simulink model "ls_legolabs"  (R2024b)
settings: Solver=FixedStepAuto  StartTime=0.0  StopTime=10.0  RelTol=1e-3  EnableMultiTasking=on
libraries: legoev3lib x14, simulink x1
settings Model: ExtModeTrigDuration=2  Creator=eline.schjerven  LastModifiedBy=seyon
settings SolverCC: PositivePriorityOrder=on
settings OptimizationCC: EnhancedBackFolding=on  PassReuseOutputArgsThreshold=0  MaxStackSize=64  OptimizeBlockOrder=speed  DifferentSizesBufferReuse=on  OptimizationCustomize=off
settings DebuggingCC: ParameterTunabilityLossMsg=error
settings HardwareCC: ProdBitPerPointer=32  ProdBitPerSizeT=32  ProdBitPerPtrDiffT=32  ProdLargestAtomicInteger=Long  ProdWordSize=32  ProdHWDeviceType=ARM Compatible->ARM 9  UseEmbeddedCoderFeatures=off  UseSimulinkCoderFeatures=off
settings SFSimCC: MATLABDynamicMemAlloc=off
settings RTWCC: Description=Embedded Coder  SystemTargetFile=ert.tlc  HardwareBoard=LEGO MINDSTORMS EV3  TLCOptions="-aInlineSetEventsForThisBaseRateFcn=TLC_FALSE -aSuppressMultiTaskScheduler=TLC_FALSE  -aRateBasedStepFcn=0"  TemplateMakefile=ert_default_tmf  Toolchain=Sourcery G++ Lite v2009q3
settings CodeAppCC: ForceParamTrailComments=on  OperatorAnnotations=on
settings ERTTargetCC: ERTCustomFileBanners=off  SupportContinuousTime=on  SupportNonInlinedSFcns=on  RemoveResetFunc=off  SupportVariableSizeSignals=on  ModelStepFunctionPrototypeControlCompliant=off  ExtModeTransport=2  ExtModeStaticAlloc=on  ExtModeMexFile=ext_xcp  ExtModeIntrfLevel=Level2 - Open  InlinedParameterPlacement=Hierarchical  DynamicArrayContainerType=coder::array

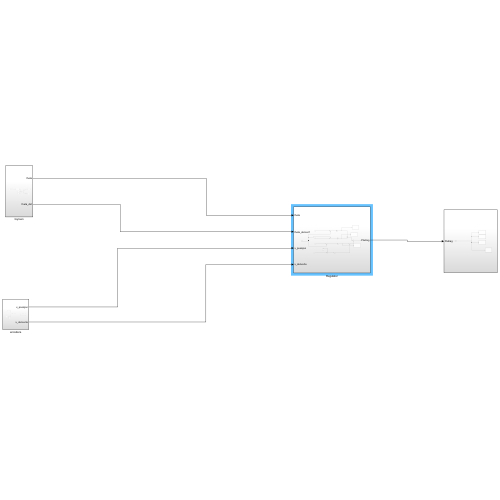
[thumbnail: Simulink's stored preview of the top-level diagram]
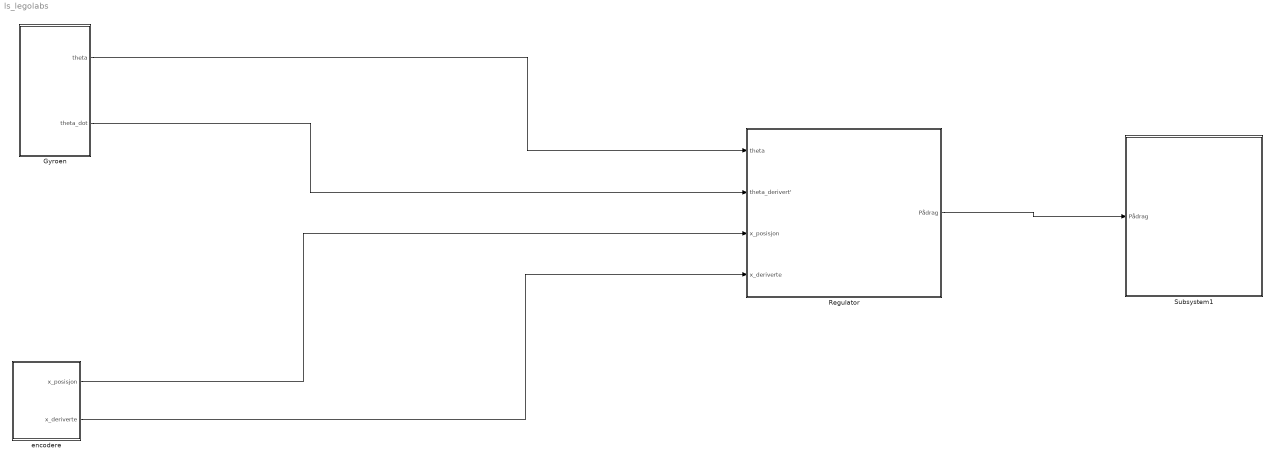
== system ls_legolabs ==
  Gyroen : Subsystem
  Regulator : Subsystem
  Subsystem1 : Subsystem
  encodere : Subsystem
  wires:
  Gyroen/2(theta_dot) -> Regulator/2(theta_derivert')
  encodere/1(x_posisjon) -> Regulator/3(x_posisjon)
  Gyroen/1(theta) -> Regulator/1(theta)
  encodere/2(x_deriverte) -> Regulator/4(x_deriverte)
  Regulator/1(Pådrag) -> Subsystem1/1(Pådrag)

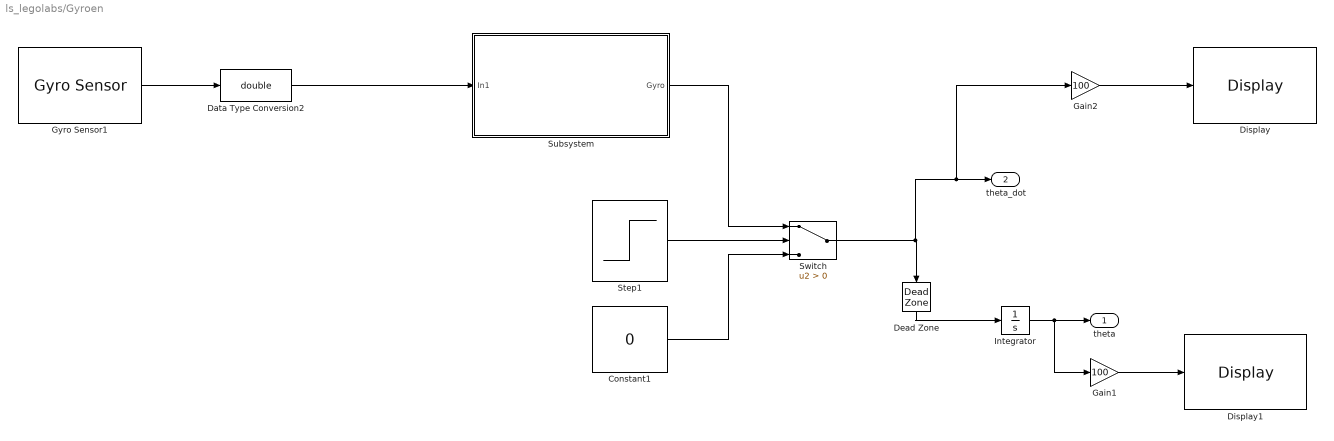
== system ls_legolabs/Gyroen ==
  Constant1 : Constant  Value=0
  Data Type Conversion2 : DataTypeConversion  OutDataTypeStr=double  SaturateOnIntegerOverflow=off  RndMeth=Floor
  Dead Zone : DeadZone  LowerValue=-1  UpperValue=1
  Display : legoev3lib/Display  slcdStr=tet_dev  slcdLine=1  slcdFormat=Decimal
  Display1 : legoev3lib/Display  slcdStr=tet  slcdLine=2  slcdFormat=Decimal
  Gain1 : Gain  Gain=100
  Gain2 : Gain  Gain=100
  Gyro Sensor1 : legoev3lib/Gyro Sensor  portNumber=2  sampleTime=0.01
  Integrator : Integrator
  Step1 : Step  Time=5  SampleTime=0
  Subsystem : Subsystem
  Switch : Switch  Criteria=u2 > Threshold  SaturateOnIntegerOverflow=off  InputSameDT=off
  theta : Outport
  theta_dot : Outport  Port=2
  wires:
  Integrator/1 -> Gain1/1, theta/1
  Gyro Sensor1/1 -> Data Type Conversion2/1
  Data Type Conversion2/1 -> Subsystem/1(In1)
  Step1/1 -> Switch/2
  Subsystem/1(Gyro) -> Switch/1
  Constant1/1 -> Switch/3
  Switch/1 -> Dead Zone/1, Gain2/1, theta_dot/1
  Gain1/1 -> Display1/1
  Gain2/1 -> Display/1
  Dead Zone/1 -> Integrator/1

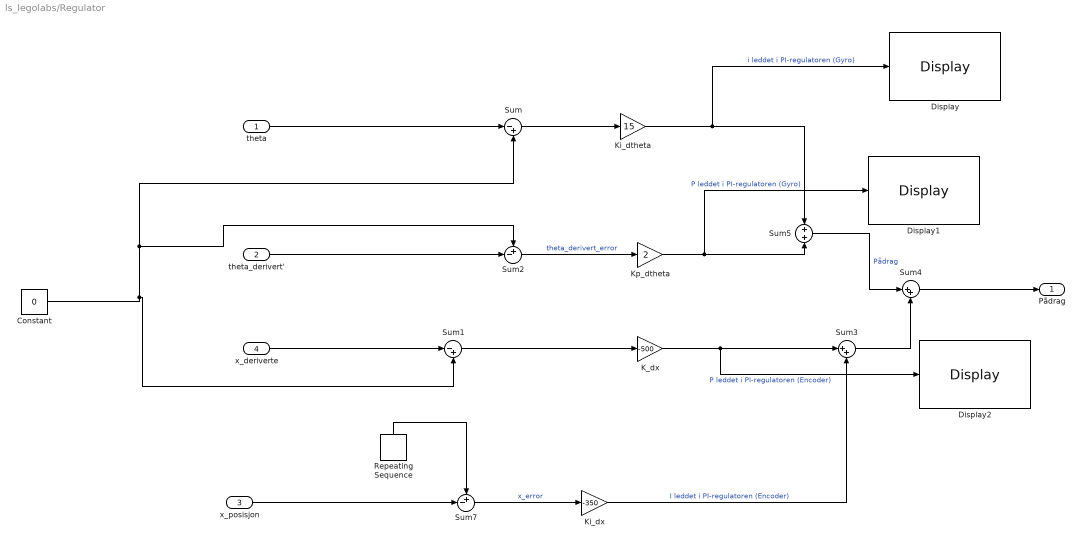
== system ls_legolabs/Regulator ==
  theta : Inport
  theta_derivert' : Inport  Port=2
  x_posisjon : Inport  Port=3
  x_deriverte : Inport  Port=4
  Constant : Constant  Value=0
  Display : legoev3lib/Display  slcdStr=Ti_I  slcdLine=9  slcdFormat=Decimal
  Display1 : legoev3lib/Display  slcdStr=Tp_dt  slcdLine=10  slcdFormat=Decimal
  Display2 : legoev3lib/Display  slcdStr=Kp_dx  slcdLine=8  slcdFormat=Decimal
  K_dx : Gain  Gain=-500
  Ki_dtheta : Gain  Gain=15
  Ki_dx : Gain  Gain=-350
  Kp_dtheta : Gain  Gain=2
  Repeating Sequence : simulink/Sources/Repeating Sequence  rep_seq_t=[0 5 7 10 12 14 16 1000]  rep_seq_y=[0 0 0.25 0.4 0.8 1.0 1.2 1.2]
  Sum : Sum  Inputs=|-+
  Sum1 : Sum  Inputs=|-+
  Sum2 : Sum  Inputs=+-|
  Sum3 : Sum  Inputs=|++
  Sum4 : Sum  Inputs=|++
  Sum5 : Sum
  Sum7 : Sum  Inputs=+-|
  Pådrag : Outport
  wires:
  Kp_dtheta/1 -> Sum5/2, Display1/1  "P leddet i PI-regulatoren (Gyro)"
  K_dx/1 -> Display2/1, Sum3/1  "P leddet i PI-regulatoren (Encoder)"
  Ki_dtheta/1 -> Display/1, Sum5/1  "i leddet i PI-regulatoren (Gyro)"
  theta_derivert'/1 -> Sum2/2
  x_posisjon/1 -> Sum7/2
  Ki_dx/1 -> Sum3/2  "I leddet i PI-regulatoren (Encoder)"
  Sum7/1 -> Ki_dx/1  "x_error"
  Sum2/1 -> Kp_dtheta/1  "theta_derivert_error"
  Sum/1 -> Ki_dtheta/1
  theta/1 -> Sum/1
  Constant/1 -> Sum1/2, Sum2/1, Sum/2
  x_deriverte/1 -> Sum1/1
  Sum1/1 -> K_dx/1
  Sum3/1 -> Sum4/2
  Sum5/1 -> Sum4/1  "Pådrag"
  Sum4/1 -> Pådrag/1
  Repeating Sequence/1 -> Sum7/1

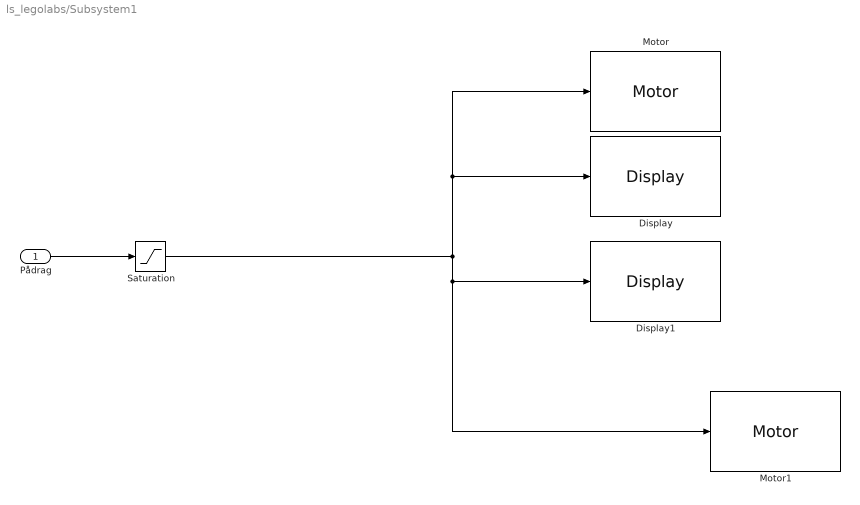
== system ls_legolabs/Subsystem1 ==
  Pådrag : Inport
  Display : legoev3lib/Display  slcdStr=Motor B  slcdLine=3  slcdFormat=Decimal
  Display1 : legoev3lib/Display  slcdStr=Motor C  slcdLine=4  slcdFormat=Decimal
  Motor : legoev3lib/Motor  sportNumber=C  sstopAction=Brake
  Motor1 : legoev3lib/Motor  sportNumber=B  sstopAction=Brake
  Saturation : Saturate  UpperLimit=100  LowerLimit=-100
  wires:
  Pådrag/1 -> Saturation/1
  Saturation/1 -> Motor1/1, Display1/1, Display/1, Motor/1

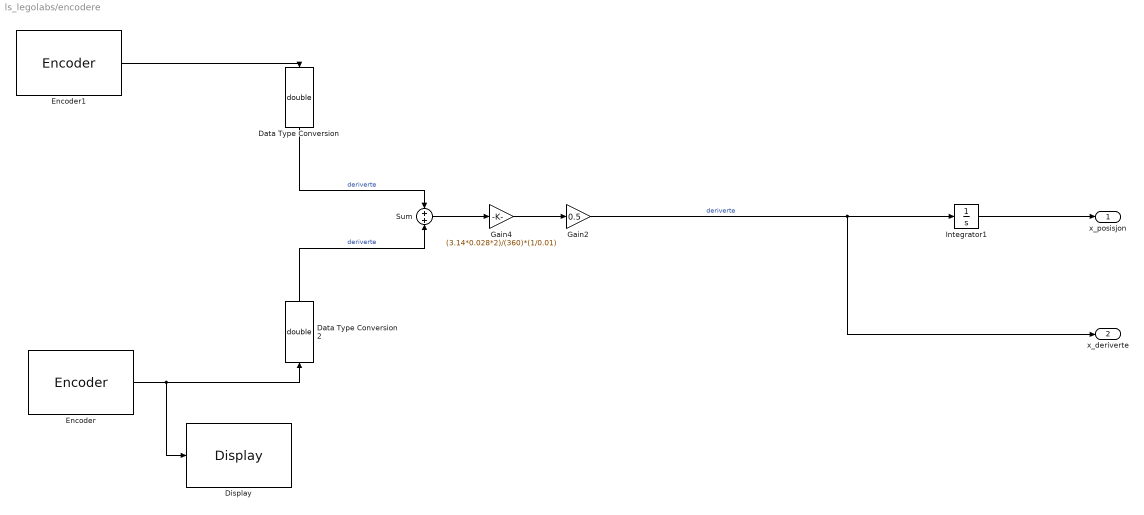
== system ls_legolabs/encodere ==
  Data Type Conversion : DataTypeConversion  OutDataTypeStr=double  SaturateOnIntegerOverflow=off  RndMeth=Floor
  Data Type Conversion2 : DataTypeConversion  OutDataTypeStr=double  SaturateOnIntegerOverflow=off  RndMeth=Floor
  Display : legoev3lib/Display  slcdStr=motoren  slcdLine=5  slcdFormat=Decimal
  Encoder : legoev3lib/Encoder  portNumber=B  opMode=Reset at each sample time  sampleTime=0.01
  Encoder1 : legoev3lib/Encoder  portNumber=C  opMode=Reset at each sample time  sampleTime=0.01
  Gain2 : Gain  Gain=0.5
  Gain4 : Gain  Gain=(3.14*0.028*2)/(360)*(1/0.01)
  Integrator1 : Integrator
  Sum : Sum
  x_posisjon : Outport
  x_deriverte : Outport  Port=2
  wires:
  Integrator1/1 -> x_posisjon/1
  Encoder/1 -> Display/1, Data Type Conversion2/1
  Encoder1/1 -> Data Type Conversion/1
  Gain2/1 -> x_deriverte/1, Integrator1/1  "deriverte"
  Sum/1 -> Gain4/1
  Data Type Conversion2/1 -> Sum/2  "deriverte"
  Data Type Conversion/1 -> Sum/1  "deriverte"
  Gain4/1 -> Gain2/1

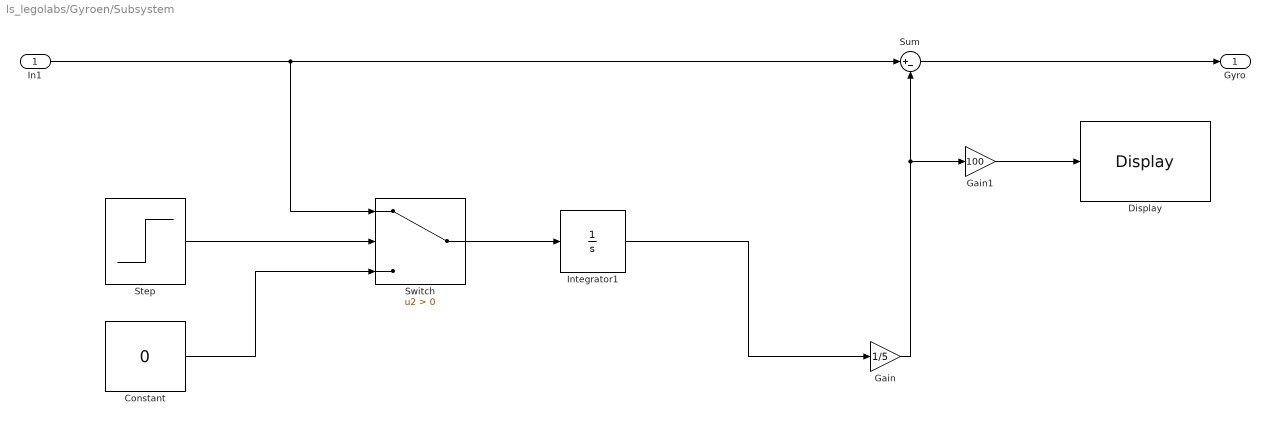
== system ls_legolabs/Gyroen/Subsystem ==
  In1 : Inport
  Constant : Constant  Value=0
  Display : legoev3lib/Display  slcdStr=bias  slcdLine=7  slcdFormat=Decimal
  Gain : Gain  Gain=1/5
  Gain1 : Gain  Gain=100
  Integrator1 : Integrator
  Step : Step  Time=5  Before=1  After=0  SampleTime=0
  Sum : Sum  Inputs=|+-
  Switch : Switch  Criteria=u2 > Threshold  SaturateOnIntegerOverflow=off  InputSameDT=off
  Gyro : Outport
  wires:
  Constant/1 -> Switch/3
  Integrator1/1 -> Gain/1
  Step/1 -> Switch/2
  Switch/1 -> Integrator1/1
  Gain/1 -> Gain1/1, Sum/2
  Sum/1 -> Gyro/1
  Gain1/1 -> Display/1
  In1/1 -> Sum/1, Switch/1
